simulink model "Copy_of_US_Image_Acquire_Trigger"  (R2018b)
settings: Solver=FixedStepAuto  StartTime=1.1  StopTime=20  FixedStep=1/30  RelTol=1e-3
undefined symbols (not defined in the file or in its folder): none, videoinput
libraries: simulink_extras x1, simulink x1, imaqlib x1, sldrtlib x1
settings Model: Creator=asgar  LastModifiedBy=asgar

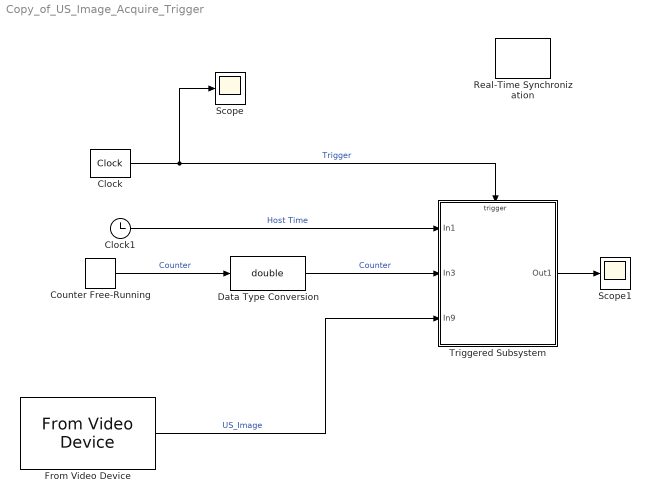
== system Copy_of_US_Image_Acquire_Trigger ==
  Clock : simulink_extras/Flip Flops/Clock  period=1
  Clock1 : Clock
  Counter Free-Running : simulink/Sources/Counter Free-Running  NumBits=32  tsamp=-1
  Data Type Conversion : DataTypeConversion  OutDataTypeStr=double
  From Video Device : imaqlib/From Video Device  DeviceMenu=winvideo 1 (Microsoft Camera Rear)  Device=winvideo 1 (DVI2USB 3.0 D2S300156)  ObjConstructor=videoinput('winvideo', 1)  VideoFormatMenu=YUY2_1280x720  VideoFormat=RGB565_1280x1024  VideoSource=input1  ROIPosition=[99 205 802 720]  EnableHWTrigger=off  TriggerConfiguration=none/none  SampleTime=1/30  OutputPortsMode=One multidimensional signal  DataType=uint8  CanDoHWTrigger=no  ReturnedColorSpace=grayscale  BlockHandle=4090.0001  ROIWidth=720  ROIHeight=802  ROIColumn=205  ROIRow=99  EngXMLPath=C:\Program Files\MATLAB\R2018b\toolbox\imaq\imaq\private  DevXMLPath=C:\ProgramData\MATLAB\SupportPackages\R2018b\toolbox\imaq\supportpackages\genericvideo\adaptor\win64  EngLibPath=C:\Program Files\MATLAB\R2018b\toolbox\imaq\imaqblks\imaqmex\win64  ColorSpace=grayscale  BayerSensorAlignment=grbg
      settings: SourceProductName=Image Acquisition Toolbox
  Real-Time Synchronization : sldrtlib/Real-Time Synchronization  SampleTime=0.3  MaxMissedTicks=8  ShowMissedTicks=on  YieldWhenWaiting=off
  Scope : Scope
  Scope1 : Scope
  Triggered Subsystem : Subsystem  TreatAsAtomicUnit=on
  wires:
  From Video Device/1 -> Triggered Subsystem/3(In9)  "US_Image"
  Clock/1 -> Scope/1, Triggered Subsystem/Trigger  "Trigger"
  Clock1/1 -> Triggered Subsystem/1(In1)  "Host Time"
  Counter Free-Running/1 -> Data Type Conversion/1  "Counter"
  Data Type Conversion/1 -> Triggered Subsystem/2(In3)  "Counter"
  Triggered Subsystem/1(Out1) -> Scope1/1

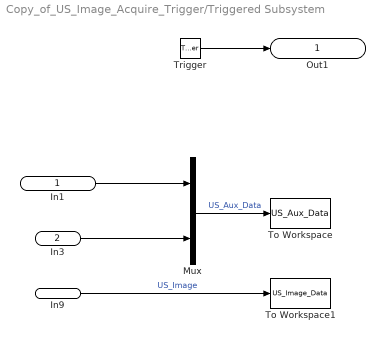
== system Copy_of_US_Image_Acquire_Trigger/Triggered Subsystem ==
  In1 : Inport
  In3 : Inport  Port=2
  In9 : Inport  Port=3
  Trigger : TriggerPort  VariantControl=Variant  ShowOutputPort=on  InitialTriggerSignalState=zero
  Mux : Mux  Inputs=2
  To Workspace : ToWorkspace  VariableName=US_Aux_Data  SampleTime=-1
      settings: Save2DSignal=2-D array (concatenate along first dimension)
  To Workspace1 : ToWorkspace  VariableName=US_Image_Data  SaveFormat=Structure With Time  SampleTime=-1
  Out1 : Outport
  wires:
  In1/1 -> Mux/1
  In3/1 -> Mux/2
  Mux/1 -> To Workspace/1  "US_Aux_Data"
  In9/1 -> To Workspace1/1  "US_Image"
  Trigger/1 -> Out1/1
